simulink model "grid_tied_control"  (Simulink 10.3)
settings: Solver=ode5  StartTime=0.0  StopTime=t_end  FixedStep=Ts  RelTol=1e-3  EnableMultiTasking=on
values from neighbouring files (symbols this model uses):
  A_r = sysd.a    [grid_tied_controller_design.m]
  B_r = sysd.b    [grid_tied_controller_design.m]
  C_r = sysd.c    [grid_tied_controller_design.m]
  CLinear = 0    [grid_tied_settings.m]
  CNLinear = 1    [grid_tied_settings.m]
  D_r = sysd.d    [grid_tied_controller_design.m]
  f = 60    [run_grid_tied.m]
  Io1_pk = 10*sqrt(2)    [grid_tied_settings.m]
  Io3_pk = Io1_pk*0.86    [grid_tied_settings.m]
  Io5_pk = Io1_pk*0.62    [grid_tied_settings.m]
  K = W/Q    [grid_tied_controller_design.m]
  K_pwm = V_cc/(2*V_sat)    (= 1)    [grid_tied_settings.m]
  T = 1/fa    (= 4.99001996008e-05)    [run_grid_tied.m]
  t_end = 2    [run_grid_tied.m]
  Ts = 1/(20*fa)    (= 2.49500998004e-06)    [run_grid_tied.m]
  u0 = V_cc/2    (= 260)    [grid_tied_settings.m]
  V_cc = 520    [grid_tied_settings.m]
  V_ma = Vo_rms*1.1    (= 139.7)    [grid_tied_settings.m]
  V_mi = Vo_rms*0.9    (= 114.3)    [grid_tied_settings.m]
libraries: powerlib_extras x2
settings Model: Creator=Projeto UPS  LastModifiedBy=gkeie
settings DataIOCC: SignalLoggingName=sigsOut
settings DebuggingCC: SaveWithParameterizedLinksMsg=none  SignalResolutionControl=TryResolveAllWithWarning  MultiTaskDSMMsg=warning  MultiTaskCondExecSysMsg=none
settings HardwareCC: TargetUnknown=on

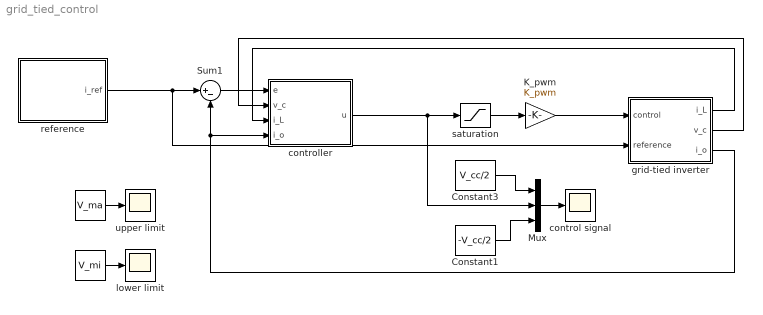
== system grid_tied_control ==
  "            " : Constant  Value=V_ma  SampleTime=-1
  "                                   " : Constant  Value=V_mi  SampleTime=-1
  " K_pwm" : Gain  Gain=K_pwm  SaturateOnIntegerOverflow=on  OutDataTypeStr=Inherit: Same as input  ParamDataTypeStr=Inherit: Same as input
  Constant1 : Constant  Value=-V_cc/2  SampleTime=-1
  Constant3 : Constant  Value=V_cc/2  SampleTime=-1
  Mux : Mux  Inputs=3
  Sum1 : Sum  Inputs=|+-  SaturateOnIntegerOverflow=on
  control signal : Scope
  controller : Subsystem
  grid-tied inverter : Subsystem
  lower limit : Scope
  reference : Subsystem
  saturation : Saturate  UpperLimit=u0  LowerLimit=-u0  LinearizeAsGain=off
  upper limit : Scope
  wires:
  Sum1/1 -> controller/1(e)
  saturation/1 -> " K_pwm"/1
  " K_pwm"/1 -> grid-tied inverter/1(control)
  Constant1/1 -> Mux/3
  "            "/1 -> upper limit/1
  Constant3/1 -> Mux/1
  controller/1(u) -> Mux/2, saturation/1
  Mux/1 -> control signal/1
  "                                   "/1 -> lower limit/1
  grid-tied inverter/2(v_c) -> controller/2(v_c)
  grid-tied inverter/3(i_o) -> controller/4(i_o), Sum1/2
  grid-tied inverter/1(i_L) -> controller/3(i_L)
  reference/1(i_ref) -> grid-tied inverter/2(reference), Sum1/1

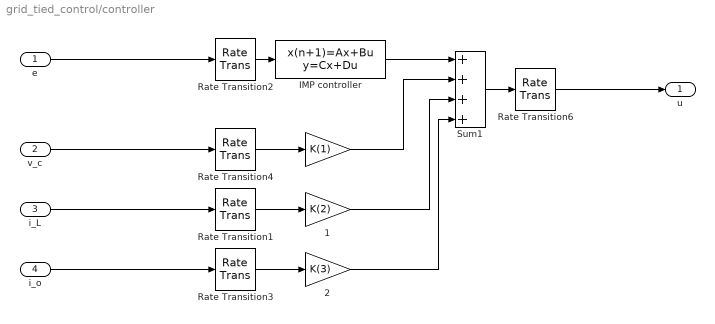
== system grid_tied_control/controller ==
  e : Inport
  v_c : Inport  Port=2
  i_L : Inport  Port=3
  i_o : Inport  Port=4
  "         " : Gain  Gain=K(1)  SaturateOnIntegerOverflow=on  OutDataTypeStr=Inherit: Same as input  ParamDataTypeStr=Inherit: Same as input
  "         1" : Gain  Gain=K(2)  SaturateOnIntegerOverflow=on  OutDataTypeStr=Inherit: Same as input  ParamDataTypeStr=Inherit: Same as input
  "         2" : Gain  Gain=K(3)  SaturateOnIntegerOverflow=on  OutDataTypeStr=Inherit: Same as input  ParamDataTypeStr=Inherit: Same as input
  IMP controller : DiscreteStateSpace  A=A_r  B=B_r  C=C_r  D=D_r  SampleTime=T
  Rate Transition{1..4,6} (5 alike) : RateTransition
  Sum1 : Sum  Inputs=++++
  u : Outport
  wires:
  "         "/1 -> Sum1/2
  e/1 -> Rate Transition2/1
  v_c/1 -> Rate Transition4/1
  Rate Transition2/1 -> IMP controller/1
  Rate Transition4/1 -> "         "/1
  Sum1/1 -> Rate Transition6/1
  Rate Transition6/1 -> u/1
  Rate Transition1/1 -> "         1"/1
  i_L/1 -> Rate Transition1/1
  i_o/1 -> Rate Transition3/1
  Rate Transition3/1 -> "         2"/1
  "         1"/1 -> Sum1/3
  "         2"/1 -> Sum1/4
  IMP controller/1 -> Sum1/1

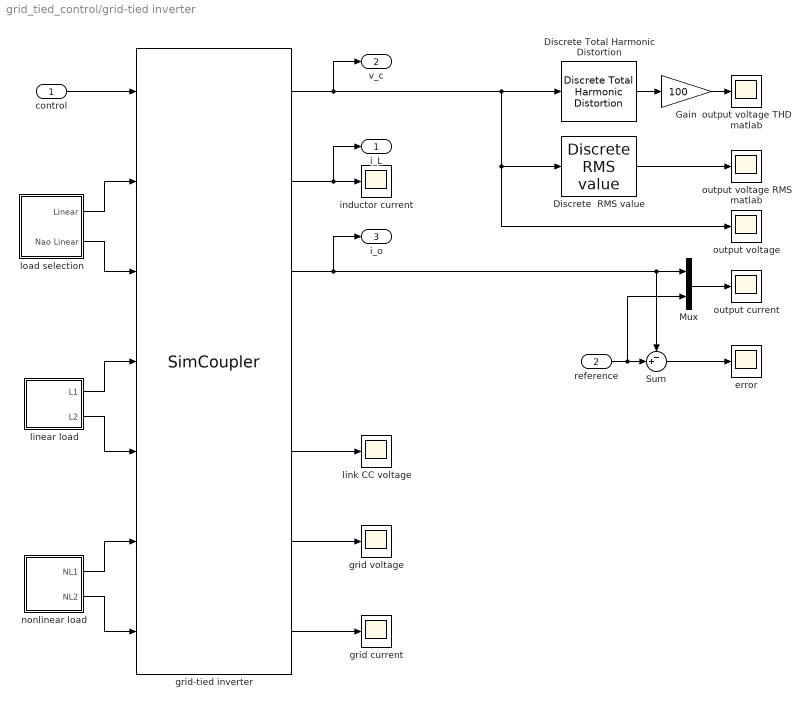
== system grid_tied_control/grid-tied inverter ==
  control : Inport
  reference : Inport  Port=2
  Discrete Total Harmonic Distortion : powerlib_extras/Discrete Measurements/Discrete Total Harmonic Distortion  Freq=f  Ts=Ts
      settings: SourceProductBaseCode=PS
  Discrete  RMS value : powerlib_extras/Discrete Measurements/Discrete  RMS value  Freq=f  Mag_Init=0  Ts=Ts
      settings: SourceProductBaseCode=PS
  Gain : Gain  Gain=100
  Mux : Mux  Inputs=2
  Sum : Sum  Inputs=-+|
  error : Scope
  grid current : Scope
  grid voltage : Scope
  grid-tied inverter : S-Function  FunctionName=SimCoupler  Parameters='C:\Users\gkeie\Documents\GitHub\grid_tied\grid_tied.psimsch'  SFunctionDeploymentMode=off  EnableBusSupport=off
      mask init:
      | c=[0:10:360]*pi/180;
      | x1=cos(c)*30; y1=sin(c)*30+20;
      | x2=cos(c)*30;y2=sin(c)*30-20;
      settings: OpenFcn=PSimDialog('PSimFileEdt','Value','Parameters');  CloseFcn=close(gcf);
      mask Display: plot(-60,-60,60,60,x1,y1,x2,y2)
  inductor current : Scope
  linear load : Subsystem
  link CC voltage : Scope
  load selection : Subsystem
  nonlinear load : Subsystem
  output current : Scope
  output voltage : Scope
  output voltage RMS matlab : Scope
  "output voltage THD matlab    " : Scope
  i_L : Outport
  v_c : Outport  Port=2
  i_o : Outport  Port=3
  wires:
  control/1 -> grid-tied inverter/1
  grid-tied inverter/1 -> v_c/1, Discrete Total Harmonic Distortion/1, output voltage/1, Discrete  RMS value/1
  grid-tied inverter/3 -> i_o/1, Mux/1, Sum/1
  grid-tied inverter/2 -> i_L/1, inductor current/1
  Discrete Total Harmonic Distortion/1 -> Gain/1
  Gain/1 -> "output voltage THD matlab    "/1
  Discrete  RMS value/1 -> output voltage RMS matlab/1
  load selection/1(Linear) -> grid-tied inverter/2
  load selection/2(Nao Linear) -> grid-tied inverter/3
  linear load/1(L1) -> grid-tied inverter/4
  linear load/2(L2) -> grid-tied inverter/5
  nonlinear load/1(NL1) -> grid-tied inverter/6
  nonlinear load/2(NL2) -> grid-tied inverter/7
  Sum/1 -> error/1
  Mux/1 -> output current/1
  grid-tied inverter/5 -> link CC voltage/1
  grid-tied inverter/7 -> grid current/1
  grid-tied inverter/6 -> grid voltage/1
  reference/1 -> Mux/2, Sum/2

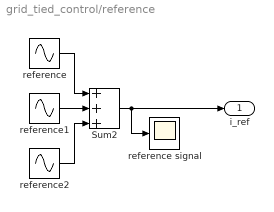
== system grid_tied_control/reference ==
  Sum2 : Sum  Inputs=+++  SaturateOnIntegerOverflow=on
  reference : Sin  Amplitude=Io1_pk  Frequency=2*pi*f  SampleTime=Ts
  reference signal : Scope
  reference1 : Sin  Amplitude=Io3_pk  Frequency=3*2*pi*f  Phase=pi  SampleTime=Ts
  reference2 : Sin  Amplitude=Io5_pk  Frequency=5*2*pi*f  SampleTime=Ts
  i_ref : Outport
  wires:
  Sum2/1 -> i_ref/1, reference signal/1
  reference/1 -> Sum2/1
  reference2/1 -> Sum2/3
  reference1/1 -> Sum2/2

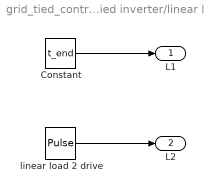
== system grid_tied_control/grid-tied inverter/linear load ==
  Constant : Constant  Value=t_end
  linear load 2 drive : DiscretePulseGenerator  PulseType=Time based  Amplitude=t_end  Period=t_end  PulseWidth=40  PhaseDelay=36/f +1/(4*f)
  L1 : Outport
  L2 : Outport  Port=2
  wires:
  Constant/1 -> L1/1
  linear load 2 drive/1 -> L2/1

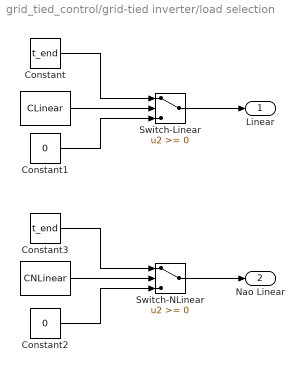
== system grid_tied_control/grid-tied inverter/load selection ==
  " " : Constant  Value=CLinear  VectorParams1D=off  OutDataTypeStr=boolean  SampleTime=-1
  "  " : Constant  Value=CNLinear  VectorParams1D=off  OutDataTypeStr=boolean  SampleTime=-1
  Constant : Constant  Value=t_end  SampleTime=-1
  Constant1 : Constant  Value=0  SampleTime=-1
  Constant2 : Constant  Value=0  SampleTime=-1
  Constant3 : Constant  Value=t_end  SampleTime=-1
  Switch-Linear : Switch
  Switch-NLinear : Switch
  Linear : Outport
  Nao Linear : Outport  Port=2
  wires:
  Switch-Linear/1 -> Linear/1
  " "/1 -> Switch-Linear/2
  Switch-NLinear/1 -> Nao Linear/1
  "  "/1 -> Switch-NLinear/2
  Constant/1 -> Switch-Linear/1
  Constant2/1 -> Switch-NLinear/3
  Constant3/1 -> Switch-NLinear/1
  Constant1/1 -> Switch-Linear/3

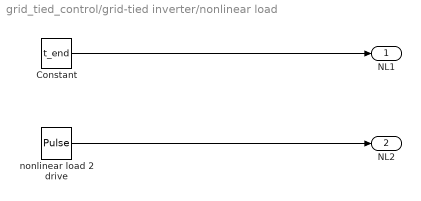
== system grid_tied_control/grid-tied inverter/nonlinear load ==
  Constant : Constant  Value=t_end
  nonlinear load 2 drive : DiscretePulseGenerator  PulseType=Time based  Amplitude=t_end  Period=t_end  PulseWidth=40  PhaseDelay=36/f +1/(4*f)
  NL1 : Outport
  NL2 : Outport  Port=2
  wires:
  Constant/1 -> NL1/1
  nonlinear load 2 drive/1 -> NL2/1
